simulink model "BSD_System"  (R2024a)
settings: Solver=FixedStepDiscrete  StartTime=0.0  StopTime=10  FixedStep=0.02  RelTol=1e-3
settings Model: Creator=pc  LastModifiedBy=pc
settings OptimizationCC: DefaultParameterBehavior=Inlined  EnhancedBackFolding=on  PassReuseOutputArgsAs=Individual arguments  ZeroExternalMemoryAtStartup=off  ZeroInternalMemoryAtStartup=off  OptimizeBlockOrder=speed  DifferentSizesBufferReuse=on  OptimizationCustomize=off  EfficientTunableParamExpr=on
settings DebuggingCC: ParameterTunabilityLossMsg=error
settings SFSimCC: MATLABDynamicMemAlloc=off
settings RTWCC: Description=AUTOSAR  SystemTargetFile=autosar.tlc  GenCodeOnly=on  TemplateMakefile=ert_default_tmf  BuildConfiguration=Faster Runs  DataTypeReplacement=CDataTypesFixedWidth
settings CodeAppCC: ForceParamTrailComments=on  IgnoreCustomStorageClasses=off  OperatorAnnotations=on  SimulinkDataObjDesc=on  SFDataObjDesc=on  InsertBlockDesc=on
settings STFCustomTargetCC: MultiwordLength=256  ParMdlRefBuildCompliant=on  CompOptLevelCompliant=on  IncludeMdlTerminateFcn=off  CombineOutputUpdateFcns=on  SuppressErrorStatus=on  ERTCustomFileBanners=on  SupportNonFinite=off  SupportComplex=off  SupportContinuousTime=off  SupportNonInlinedSFcns=off  RemoveResetFunc=on  MATLABClassNameForMDSCustomization=Simulink.SoftwareTarget.ERTCustomization  AutosarCompliant=on  GRTInterface=off  LookupTableObjectStructAxisOrder=2,1,3,4,...  LUTObjectStructOrderEvenSpacing=Size,Table,Breakpoints  SystemTargetFile=autosar.tlc
settings ERTTargetCC: TargetLangStandard=C99 (ISO)  ConcurrentExecutionCompliant=off  IncludeMdlTerminateFcn=off  SuppressErrorStatus=on  SupportNonFinite=off  SupportComplex=off  ModelStepFunctionPrototypeControlCompliant=off  CPPClassGenCompliant=off  AutosarCompliant=on  LookupTableObjectStructAxisOrder=2,1,3,4,...  LUTObjectStructOrderEvenSpacing=Size,Table,Breakpoints  InlinedParameterPlacement=NonHierarchical  ERTCustomFileTemplate=example_file_process.tlc  BooleanTrueId=TRUE  BooleanFalseId=FALSE

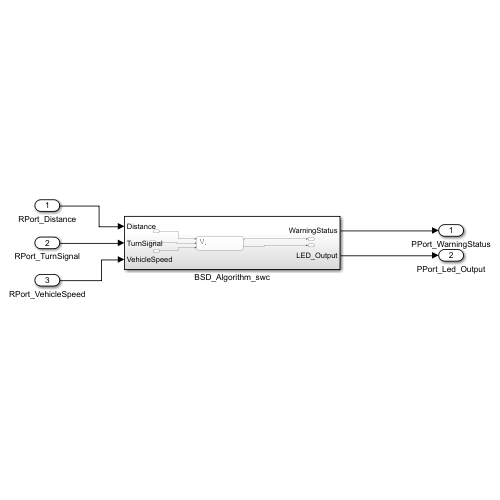
[thumbnail: Simulink's stored preview of the top-level diagram]
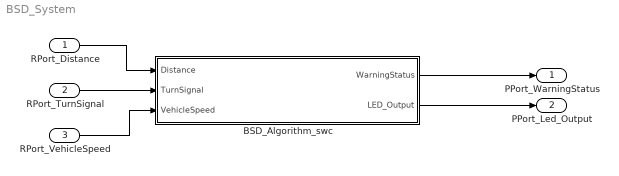
== system BSD_System ==
  RPort_Distance : Inport
  RPort_TurnSignal : Inport  Port=2
  RPort_VehicleSpeed : Inport  Port=3
  BSD_Algorithm_swc : Subsystem
  PPort_WarningStatus : Outport
  PPort_Led_Output : Outport  Port=2
  wires:
  RPort_VehicleSpeed/1 -> BSD_Algorithm_swc/3(VehicleSpeed)
  RPort_TurnSignal/1 -> BSD_Algorithm_swc/2(TurnSignal)
  RPort_Distance/1 -> BSD_Algorithm_swc/1(Distance)
  BSD_Algorithm_swc/1(WarningStatus) -> PPort_WarningStatus/1
  BSD_Algorithm_swc/2(LED_Output) -> PPort_Led_Output/1

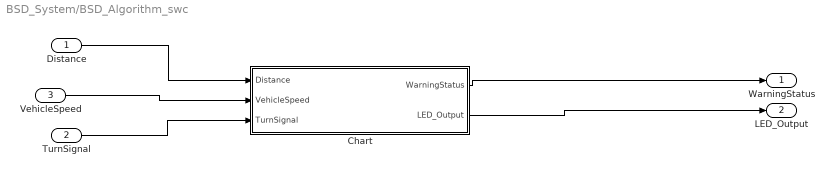
== system BSD_System/BSD_Algorithm_swc ==
  Distance : Inport  OutDataTypeStr=single  Unit=m
  TurnSignal : Inport  Port=2  OutDataTypeStr=uint8
  VehicleSpeed : Inport  Port=3  OutDataTypeStr=single  Unit=km/h
  Chart : Stateflow chart  TreatAsAtomicUnit=on
  WarningStatus : Outport  OutDataTypeStr=uint8
  LED_Output : Outport  Port=2  OutDataTypeStr=uint8
  wires:
  Distance/1 -> Chart/1(Distance)
  TurnSignal/1 -> Chart/3(TurnSignal)
  VehicleSpeed/1 -> Chart/2(VehicleSpeed)
  Chart/1(WarningStatus) -> WarningStatus/1
  Chart/2(LED_Output) -> LED_Output/1

== stateflow chart BSD_System/BSD_Algorithm_swc/Chart ==
  note: // Define outputs
      | output uint8 WarningStatus;
      | output uint8 LED_Output;
      |
      | // Define inputs
      | input single Distance;
      | input uint8 TurnSignal;
      | input single VehicleSpeed;
  state WARNING
    entry:WarningStatus = 1;
    LED_Output = 1;
  state CLEAR
    entry:WarningStatus = 0;
    LED_Output = 0;
  state ALERT
    entry:WarningStatus = 2;
    LED_Output = 1;
  CLEAR -> WARNING : [Distance < 3.0 && VehicleSpeed > 10]
  (default) -> CLEAR
  WARNING -> CLEAR [order 1] : [Distance >= 3.0]
  ALERT -> WARNING [order 1] : [TurnSignal == 0]
  WARNING -> ALERT [order 2] : [Distance < 3.0 && TurnSignal > 0]
  ALERT -> CLEAR [order 2] : [Distance >= 3.0]
  data: Distance input; VehicleSpeed input; TurnSignal input; WarningStatus output uint8; LED_Output output uint8
